simulink model "model_adaptive_robust"  (R2022b)
settings: Solver=VariableStepAuto  StartTime=0.0  StopTime=1000000  MaxStep=1e-1  RelTol=1e-3
undefined symbols (not defined in the file): A, A0, b, C, gamma, k0, k1, theta
settings Model: SimulationMode=rapid-accelerator  Creator=deniskirbaba  LastModifiedBy=R1303-We2-5-Stud
settings OptimizationCC: ReuseModelBlockBuffer=on

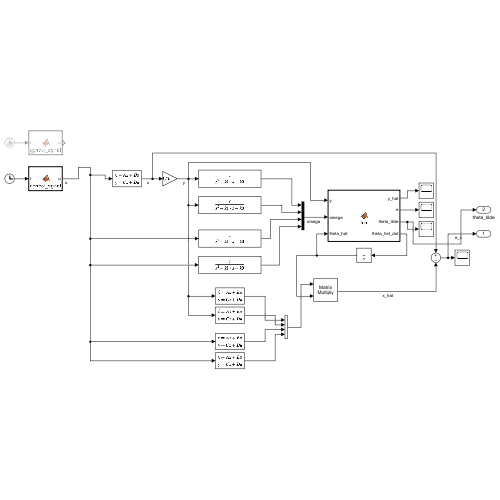
[thumbnail: Simulink's stored preview of the top-level diagram]
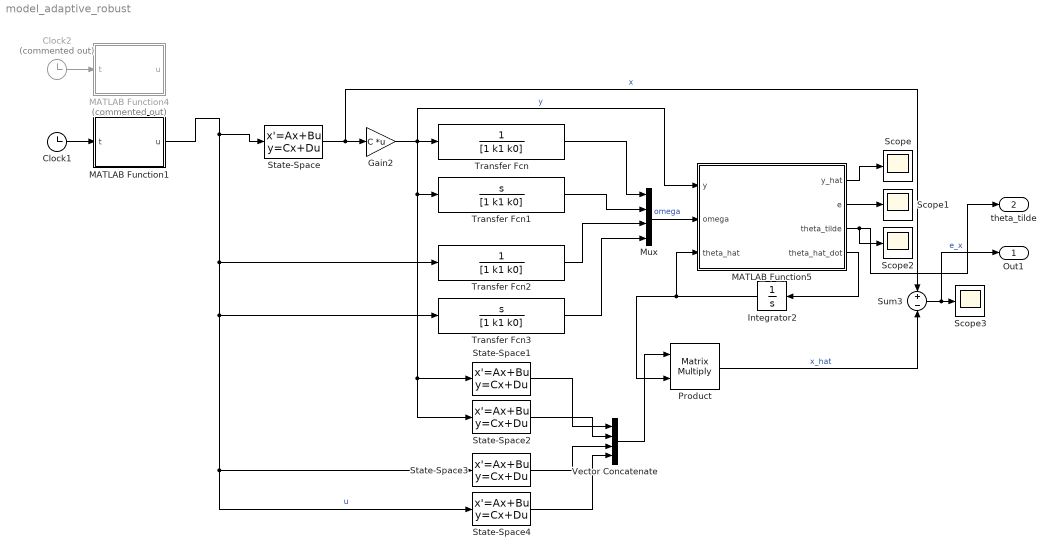
== system model_adaptive_robust ==
  Clock1 : Clock
  Clock2 : Clock  Commented=on
  Gain2 : Gain  Gain=C  Multiplication=Matrix(K*u)
  Integrator2 : Integrator  InitialCondition=[0;0;0;0]
  MATLAB Function1 : MATLAB Function  TreatAsAtomicUnit=on
  MATLAB Function4 : MATLAB Function  Commented=on  TreatAsAtomicUnit=on
  MATLAB Function5 : MATLAB Function  TreatAsAtomicUnit=on
  Mux : Mux
  Product : Product  Multiplication=Matrix(*)
  Scope{,1..3} (4 alike) : Scope
  State-Space : StateSpace  A=A  B=b  C=eye(2)  D=[0;0]  InitialCondition=[0;0]
  State-Space1 : StateSpace  A=A0  B=[0; 1]  C=eye(2)  D=[0;0]  InitialCondition=[0;0]
  State-Space2 : StateSpace  A=A0  B=[1; 0]  C=eye(2)  D=[0;0]  InitialCondition=[0;0]
  State-Space3 : StateSpace  A=A0  B=[0; 1]  C=eye(2)  D=[0;0]  InitialCondition=[0;0]
  State-Space4 : StateSpace  A=A0  B=[1; 0]  C=eye(2)  D=[0;0]  InitialCondition=[0;0]
  Sum3 : Sum  Inputs=+-
  Transfer Fcn : TransferFcn  Denominator=[1 k1 k0]
  Transfer Fcn1 : TransferFcn  Numerator=[1 0]  Denominator=[1 k1 k0]
  Transfer Fcn2 : TransferFcn  Denominator=[1 k1 k0]
  Transfer Fcn3 : TransferFcn  Numerator=[1 0]  Denominator=[1 k1 k0]
  Vector Concatenate : Concatenate  NumInputs=4  Mode=Multidimensional array  ConcatenateDimension=2
  Out1 : Outport
  theta_tilde : Outport  Port=2
  wires:
  Clock2/1 -> MATLAB Function4/1(t)
  MATLAB Function1/1(u) -> State-Space4/1, State-Space3/1, Transfer Fcn3/1, Transfer Fcn2/1, State-Space/1  "u"
  State-Space/1 -> Sum3/1, Gain2/1  "x"
  Gain2/1 -> State-Space2/1, State-Space1/1, Transfer Fcn1/1, MATLAB Function5/1(y), Transfer Fcn/1  "y"
  Transfer Fcn3/1 -> Mux/4
  Transfer Fcn2/1 -> Mux/3
  Transfer Fcn1/1 -> Mux/2
  Transfer Fcn/1 -> Mux/1
  Mux/1 -> MATLAB Function5/2(omega)  "omega"
  MATLAB Function5/4(theta_hat_dot) -> Integrator2/1
  Integrator2/1 -> Product/2, MATLAB Function5/3(theta_hat)
  State-Space1/1 -> Vector Concatenate/1
  State-Space2/1 -> Vector Concatenate/2
  State-Space3/1 -> Vector Concatenate/3
  State-Space4/1 -> Vector Concatenate/4
  Vector Concatenate/1 -> Product/1
  MATLAB Function5/1(y_hat) -> Scope/1
  MATLAB Function5/2(e) -> Scope1/1
  MATLAB Function5/3(theta_tilde) -> theta_tilde/1, Scope2/1
  Product/1 -> Sum3/2  "x_hat"
  Sum3/1 -> Out1/1, Scope3/1  "e_x"
  Clock1/1 -> MATLAB Function1/1(t)

== matlab function model_adaptive_robust/MATLAB Function1 ==
  data: t input; u output
function u = control_signal(t)
    u = 10*sin(t) + 5*cos(2*t) + 4*cos(4*t) + 3*cos(8*t);
end

== matlab function model_adaptive_robust/MATLAB Function4 ==
  data: t input; u output
function u = control_signal(t)
    u = sin(t) + 0.5*cos(2*t);
end

== matlab function model_adaptive_robust/MATLAB Function5 ==
  data: y input; omega input; theta_hat input; y_hat output; theta parameter; e output; theta_tilde output; theta_hat_dot output; gamma parameter
function [y_hat, e, theta_tilde, theta_hat_dot] = fcn(y, omega, theta_hat, theta, gamma)
    y_hat = theta_hat'*omega;
    e = y - y_hat;
    theta_hat_dot = gamma*omega*e;
    theta_tilde = theta-theta_hat;
end
